simulink model "b1int_solver_var"  (R2018b)
settings: Solver=VariableStepAuto  StartTime=0.0  StopTime=3.5  FixedStep=0.5  RelTol=1e-3  EnableMultiTasking=on
StopFcn:
  | b1erg=[tout,yout]
  | clear tout  yout
settings Model: Creator=The MathWorks, Inc.  LastModifiedBy=Reichl
settings DataIOCC: LimitDataPoints=on  SaveFormat=Array
settings OptimizationCC: ExpressionDepthLimit=2147483647  LifeSpan=inf
settings DebuggingCC: UnderspecifiedInitializationDetection=Classic  MergeDetectMultiDrivingBlocksExec=none  InheritedTsInSrcMsg=none  FcnCallInpInsideContextMsg=warning  StateNameClashWarn=warning  SFUnexpectedBacktrackingDiag=warning  SFNoUnconditionalDefaultTransitionDiag=warning  SFExecutionAtInitializationDiag=none
settings HardwareCC: ProdBitPerPointer=32  ProdBitPerSizeT=32  ProdBitPerPtrDiffT=32  ProdLargestAtomicFloat=None  ProdIntDivRoundTo=Undefined  ProdEndianess=Unspecified  ProdWordSize=32  ProdHWDeviceType=32-bit Generic
settings ModelReferenceCC: PropagateSignalLabelsOutOfModel=off
settings SFSimCC: SimUseLocalCustomCode=off
settings RTWCC: RTWUseLocalCustomCode=off
settings CodeAppCC: StateflowObjectComments=on
settings GRTTargetCC: TargetLangStandard=C89/C90 (ANSI)  GeneratePreprocessorConditionals=Disable all  CombineOutputUpdateFcns=off  GRTInterface=on
settings ConfigComp: CovMetricSettings=dw  CovHtmlReporting=on  CovSaveCumulativeToWorkspaceVar=on  CovSaveSingleToWorkspaceVar=on  CovExternalEMLEnable=off

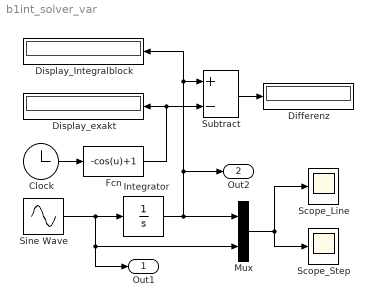
== system b1int_solver_var ==
  Clock : Clock
  Differenz : Display
      settings: Format=short_e
  Display_Integralblock : Display
  Display_exakt : Display
  Fcn : Fcn  Expr=-cos(u)+1
  Integrator : Integrator
  Mux : Mux  Inputs=2
  Scope_Line : Scope
  Scope_Step : Scope
  Sine Wave : Sin  SampleTime=0
  Subtract : Sum  Inputs=+-
  Out1 : Outport
  Out2 : Outport  Port=2
  wires:
  Sine Wave/1 -> Integrator/1, Out1/1, Mux/2
  Integrator/1 -> Out2/1, Display_Integralblock/1, Subtract/1, Mux/1
  Mux/1 -> Scope_Line/1, Scope_Step/1
  Fcn/1 -> Subtract/2, Display_exakt/1
  Clock/1 -> Fcn/1
  Subtract/1 -> Differenz/1
